simulink model "Liquid_Level_Control_Digital_1_24_RoaaTareq"  (R2022a)
settings: Solver=VariableStepAuto  StartTime=0.0  StopTime=10  RelTol=1e-3
settings Model: Creator=hp  LastModifiedBy=hp

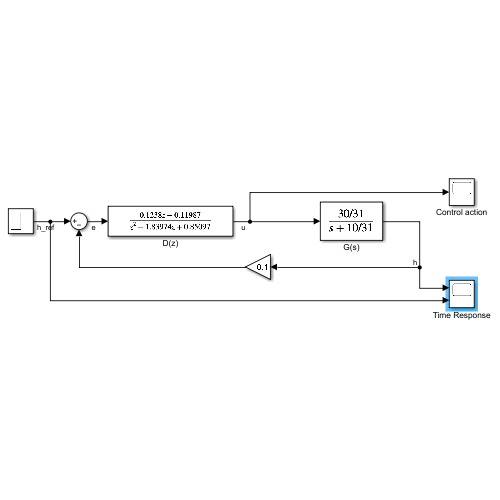
[thumbnail: Simulink's stored preview of the top-level diagram]
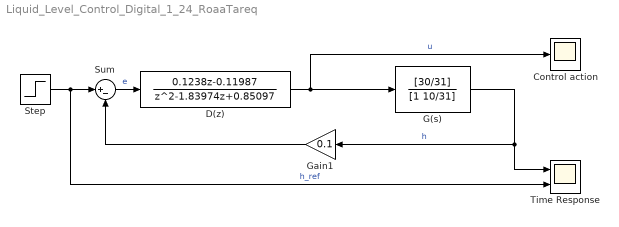
== system Liquid_Level_Control_Digital_1_24_RoaaTareq ==
  Control action : Scope
  D(z) : DiscreteTransferFcn  Numerator=[0.1238 -0.11987]  Denominator=[1 -1.83974 0.85097]  SampleTime=0.1
  G(s) : TransferFcn  Numerator=[30/31]  Denominator=[1 10/31]
  Gain1 : Gain  Gain=0.1
  Step : Step  Time=0  After=50  SampleTime=0
  Sum : Sum  Inputs=|+-
  Time Response : Scope  NumInputPorts=2
  wires:
  D(z)/1 -> G(s)/1, Control action/1  "u"
  G(s)/1 -> Time Response/1, Gain1/1  "h"
  Gain1/1 -> Sum/2
  Step/1 -> Time Response/2, Sum/1  "h_ref"
  Sum/1 -> D(z)/1  "e"
